simulink library "spin"  (R2016b)
settings: Solver=VariableStepAuto  StartTime=0.0  StopTime=10.0  RelTol=1e-3
libraries: aerolibutil x1
settings Model: Creator=nzhao  LastModifiedBy=nzhao

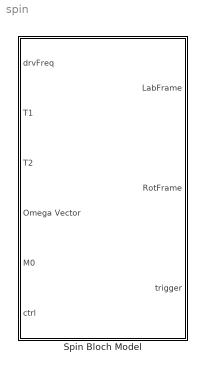
== system spin ==
  Spin Bloch Model : Subsystem

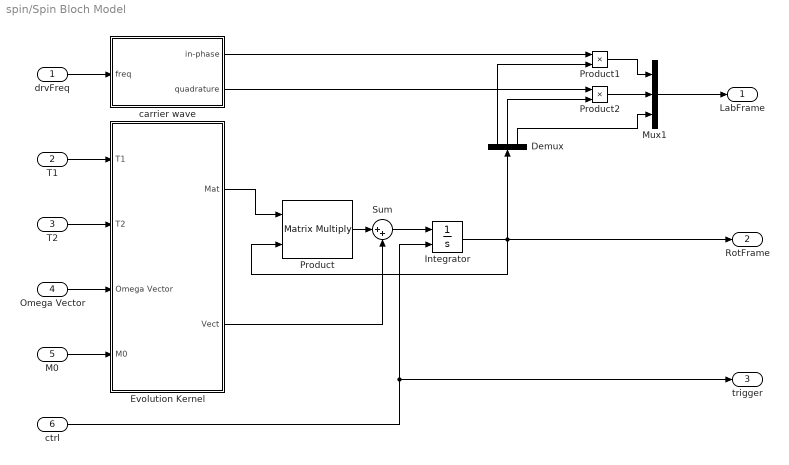
== system spin/Spin Bloch Model ==
  drvFreq : Inport
  T1 : Inport  Port=2
  T2 : Inport  Port=3
  Omega Vector : Inport  Port=4
  M0 : Inport  Port=5
  ctrl : Inport  Port=6
  Demux : Demux  Outputs=3
  Evolution Kernel : Subsystem
  Integrator : Integrator  ExternalReset=rising
  Mux1 : Mux  Inputs=3
  Product : Product  Multiplication=Matrix(*)
  Product1 : Product
  Product2 : Product
  Sum : Sum  Inputs=|++
  carrier wave : Subsystem
  LabFrame : Outport
  RotFrame : Outport  Port=2
  trigger : Outport  Port=3
  wires:
  carrier wave/2(quadrature) -> Product2/1
  Demux/3 -> Mux1/3
  Demux/2 -> Product2/2
  Product2/1 -> Mux1/2
  Mux1/1 -> LabFrame/1
  Demux/1 -> Product1/2
  Product1/1 -> Mux1/1
  drvFreq/1 -> carrier wave/1(freq)
  carrier wave/1(in-phase) -> Product1/1
  Evolution Kernel/1(Mat) -> Product/1
  Evolution Kernel/2(Vect) -> Sum/2
  T1/1 -> Evolution Kernel/1(T1)
  T2/1 -> Evolution Kernel/2(T2)
  Omega Vector/1 -> Evolution Kernel/3(Omega Vector)
  M0/1 -> Evolution Kernel/4(M0)
  Product/1 -> Sum/1
  Sum/1 -> Integrator/1
  Integrator/1 -> RotFrame/1, Product/2, Demux/1
  ctrl/1 -> Integrator/2, trigger/1

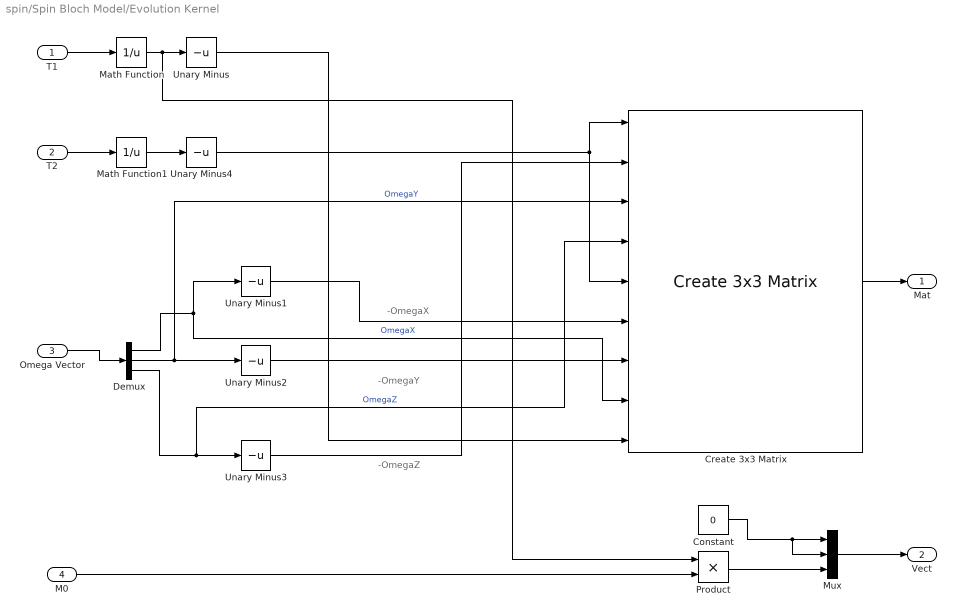
== system spin/Spin Bloch Model/Evolution Kernel ==
  note: -OmegaX
  note: -OmegaY
  note: -OmegaZ
  T1 : Inport
  T2 : Inport  Port=2
  Omega Vector : Inport  Port=3
  M0 : Inport  Port=4
  Constant : Constant  Value=0
  Create 3x3 Matrix : aerolibutil/Create 3x3 Matrix
  Demux : Demux  Outputs=3
  Math Function : Math  Operator=reciprocal  SaturateOnIntegerOverflow=on
  Math Function1 : Math  Operator=reciprocal  SaturateOnIntegerOverflow=on
  Mux : Mux  Inputs=3
  Product : Product
  Unary Minus{,1..4} (5 alike) : UnaryMinus
  Mat : Outport
  Vect : Outport  Port=2
  wires:
  Mux/1 -> Vect/1
  Omega Vector/1 -> Demux/1
  Unary Minus/1 -> Create 3x3 Matrix/9
  Product/1 -> Mux/3
  Math Function1/1 -> Unary Minus4/1
  T2/1 -> Math Function1/1
  Unary Minus2/1 -> Create 3x3 Matrix/7
  Create 3x3 Matrix/1 -> Mat/1
  M0/1 -> Product/2
  Constant/1 -> Mux/2, Mux/1
  Math Function/1 -> Product/1, Unary Minus/1
  Demux/2 -> Create 3x3 Matrix/3, Unary Minus2/1  "OmegaY"
  Demux/1 -> Unary Minus1/1, Create 3x3 Matrix/8  "OmegaX"
  Unary Minus4/1 -> Create 3x3 Matrix/1, Create 3x3 Matrix/5
  Demux/3 -> Unary Minus3/1, Create 3x3 Matrix/4  "OmegaZ"
  Unary Minus3/1 -> Create 3x3 Matrix/2
  Unary Minus1/1 -> Create 3x3 Matrix/6
  T1/1 -> Math Function/1

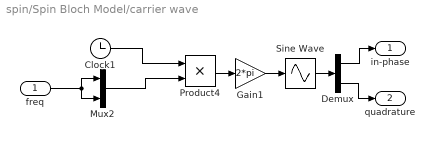
== system spin/Spin Bloch Model/carrier wave ==
  freq : Inport
  Clock1 : Clock
  Demux : Demux  Outputs=2
  Gain1 : Gain  Gain=2*pi
  Mux2 : Mux  Inputs=2
  Product4 : Product
  Sine Wave : Sin  TimeSource=Use external signal  Phase=[0 pi/2]  SampleTime=0
  in-phase : Outport
  quadrature : Outport  Port=2
  wires:
  Sine Wave/1 -> Demux/1
  Mux2/1 -> Product4/2
  Product4/1 -> Gain1/1
  Gain1/1 -> Sine Wave/1
  Clock1/1 -> Product4/1
  freq/1 -> Mux2/1, Mux2/2
  Demux/1 -> in-phase/1
  Demux/2 -> quadrature/1
